simulink model "Force_Cotrol_Test"  (R2020a)
settings: Solver=FixedStepAuto  StartTime=0.0  StopTime=inf  FixedStep=0.002  RelTol=1e-3  EnableMultiTasking=on
libraries: xpcethercatlib x8, slrtlib x6, simulink x2, simulink_extras x1
settings Model: xpc_rtwmakecfg_data=_xpcethercatlib_  SimulationMode=external  Creator=Ali  LastModifiedBy=Ali
settings SolverCC: ConcurrentTasks=on  AutoInsertRateTranBlk=on
settings DataIOCC: SaveFormat=StructureWithTime
settings OptimizationCC: BlockReduction=off  OptimizeBlockIOStorage=off
settings HardwareCC: ProdBitPerPointer=32  ProdBitPerSizeT=32  ProdBitPerPtrDiffT=32  ProdLargestAtomicFloat=None  ProdWordSize=32  ProdLongLongMode=on  ProdHWDeviceType=Generic->32-bit x86 compatible
settings RTWCC: Description=Simulink Real-Time  SystemTargetFile=slrt.tlc  TemplateMakefile=slrt_default_tmf  CodeExecutionProfiling=on  CodeProfilingInstrumentation=detailed  RTWCompilerOptimization=on
settings SimulinkRealTimeCC: SupportVariableSizeSignals=on  xPCConcurrentTasks=on

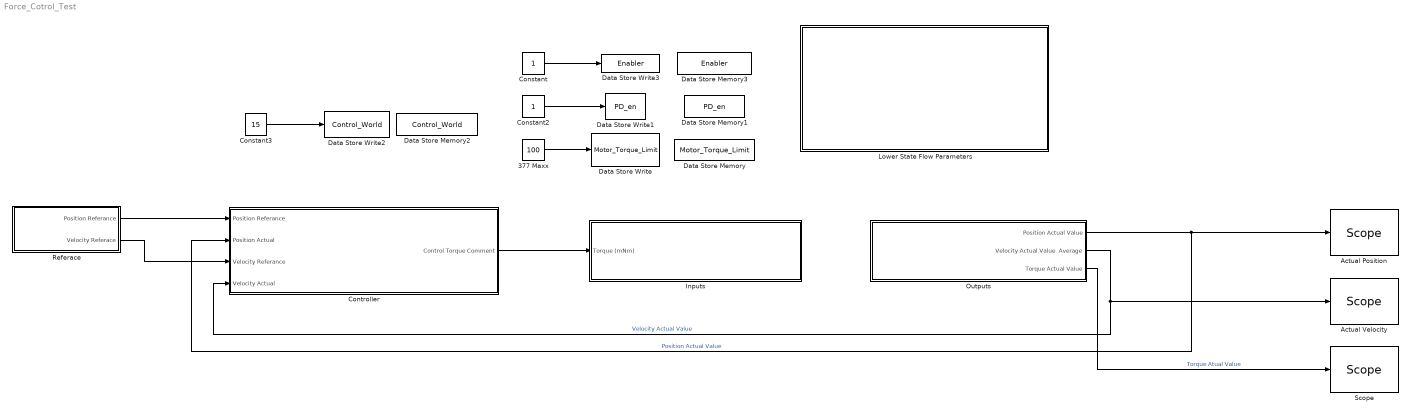
== system Force_Cotrol_Test ==
  377 Maxx : Constant  Value=100
  "Actual Position " : slrtlib/Displays and Logging/Scope   scopeno=4  scopetype=Target  autostart=on  viewmode=Graphical redraw  formatstr='%15.6f'  grid=on  ylimits=[0,0]  nosamples=250  noprepostsamples=0  interleave=1  triggermode=FreeRun  triggersignal=1  trigsignalfromport=off  triggerlevel=0.0  triggerslope=Either  triggerscope=1  triggersample=0  filename=data.dat  mode=Lazy  writesize=512  autorestart=off  dynamicfilemode=off  maxwritefilesize=512*1024^2
  Actual Velocity : slrtlib/Displays and Logging/Scope   scopeno=5  scopetype=Target  autostart=on  viewmode=Graphical redraw  formatstr='%15.6f'  grid=on  ylimits=[0,0]  nosamples=250  noprepostsamples=0  interleave=1  triggermode=FreeRun  triggersignal=1  trigsignalfromport=off  triggerlevel=0.0  triggerslope=Either  triggerscope=1  triggersample=0  filename=data.dat  mode=Lazy  writesize=512  autorestart=off  dynamicfilemode=off  maxwritefilesize=512*1024^2
  Constant : Constant
  Constant2 : Constant
  Constant3 : Constant  Value=15
  Controller : Subsystem
  Data Store Memory : DataStoreMemory  DataStoreName=Motor_Torque_Limit  ReadBeforeWriteMsg=warning  WriteAfterWriteMsg=warning  WriteAfterReadMsg=warning  ShowAdditionalParam=off
  Data Store Memory1 : DataStoreMemory  DataStoreName=PD_en  ReadBeforeWriteMsg=warning  WriteAfterWriteMsg=warning  WriteAfterReadMsg=warning  ShowAdditionalParam=off
  Data Store Memory2 : DataStoreMemory  DataStoreName=Control_World  ReadBeforeWriteMsg=warning  WriteAfterWriteMsg=warning  WriteAfterReadMsg=warning  ShowAdditionalParam=off
  Data Store Memory3 : DataStoreMemory  DataStoreName=Enabler  ReadBeforeWriteMsg=warning  WriteAfterWriteMsg=warning  WriteAfterReadMsg=warning  ShowAdditionalParam=off
  Data Store Write : DataStoreWrite  DataStoreName=Motor_Torque_Limit
  Data Store Write1 : DataStoreWrite  DataStoreName=PD_en
  Data Store Write2 : DataStoreWrite  DataStoreName=Control_World
  Data Store Write3 : DataStoreWrite  DataStoreName=Enabler
  Inputs : Subsystem
  Lower State Flow Parameters : Subsystem
  Outputs : Subsystem
  Referace : Subsystem
  "Scope " : slrtlib/Displays and Logging/Scope   scopeno=6  scopetype=Target  autostart=on  viewmode=Graphical redraw  formatstr='%15.6f'  grid=on  ylimits=[0,0]  nosamples=250  noprepostsamples=0  interleave=1  triggermode=FreeRun  triggersignal=1  trigsignalfromport=off  triggerlevel=0.0  triggerslope=Either  triggerscope=1  triggersample=0  filename=data.dat  mode=Lazy  writesize=512  autorestart=off  dynamicfilemode=off  maxwritefilesize=512*1024^2
  wires:
  377 Maxx/1 -> Data Store Write/1
  Outputs/1(Position Actual Value) -> Controller/2("Position Actual "), "Actual Position "/1  "Position Actual Value"
  Outputs/2(Velocity Actual Value  Average) -> Controller/4(Velocity Actual), Actual Velocity/1  "Velocity Actual Value"
  Referace/1(Position Referance) -> Controller/1(Position Referance)
  Referace/2(Velocity Referace) -> Controller/3(Velocity Referance)
  Constant2/1 -> Data Store Write1/1
  Controller/1(Control Torque Comment) -> Inputs/1(Torque (mNm))
  Constant3/1 -> Data Store Write2/1
  Constant/1 -> Data Store Write3/1
  Outputs/3(Torque Actual Value) -> "Scope "/1  "Torque Atual Value"

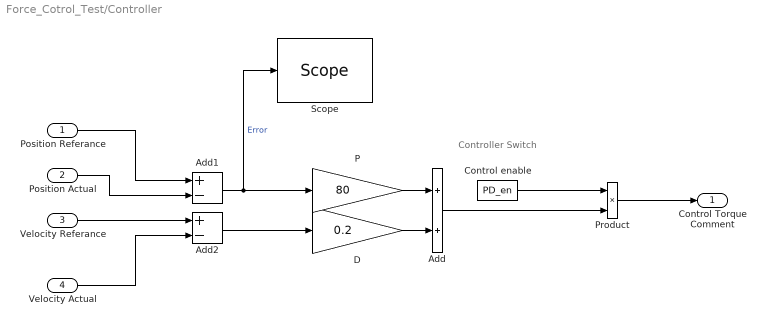
== system Force_Cotrol_Test/Controller ==
  note: Controller Switch
  Position Referance : Inport
  "Position Actual " : Inport  Port=2
  Velocity Referance : Inport  Port=3
  Velocity Actual : Inport  Port=4
  Add : Sum
  Add1 : Sum  Inputs=+-
  Add2 : Sum  Inputs=+-
  Control enable : DataStoreRead  DataStoreName=PD_en
  D : Gain  Gain=0.2
  P : Gain  Gain=80
  Product : Product
  "Scope " : slrtlib/Displays and Logging/Scope   scopeno=2  scopetype=Target  autostart=on  viewmode=Graphical redraw  formatstr='%15.6f'  grid=on  ylimits=[0,0]  nosamples=250  noprepostsamples=0  interleave=1  triggermode=FreeRun  triggersignal=1  trigsignalfromport=off  triggerlevel=0.0  triggerslope=Either  triggerscope=1  triggersample=0  filename=data.dat  mode=Lazy  writesize=512  autorestart=off  dynamicfilemode=off  maxwritefilesize=512*1024^2
  Control Torque Comment : Outport
  wires:
  D/1 -> Add/2
  Add2/1 -> D/1
  Product/1 -> Control Torque Comment/1
  Add1/1 -> "Scope "/1, P/1  "Error"
  Add/1 -> Product/2
  Velocity Referance/1 -> Add2/1
  "Position Actual "/1 -> Add1/2
  Position Referance/1 -> Add1/1
  P/1 -> Add/1
  Velocity Actual/1 -> Add2/2
  Control enable/1 -> Product/1

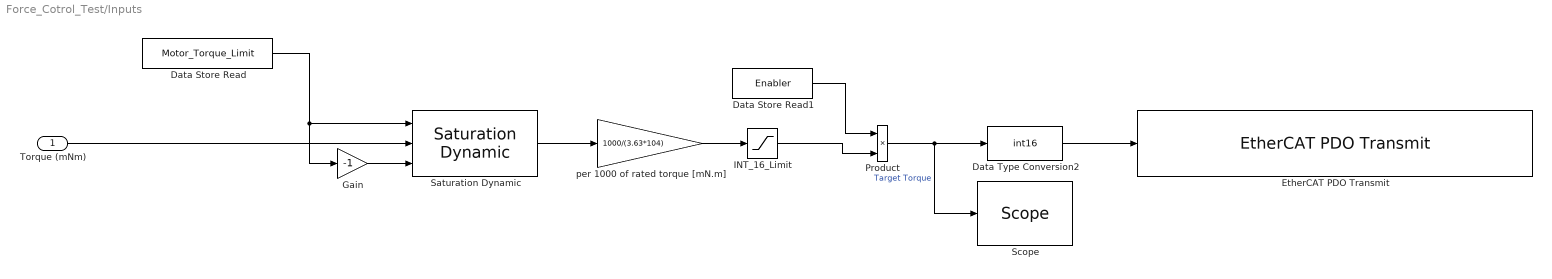
== system Force_Cotrol_Test/Inputs ==
  Torque (mNm) : Inport
  Data Store Read : DataStoreRead  DataStoreName=Motor_Torque_Limit
  Data Store Read1 : DataStoreRead  DataStoreName=Enabler
  Data Type Conversion2 : DataTypeConversion  OutDataTypeStr=int16
  "EtherCAT PDO Transmit " : xpcethercatlib/EtherCAT PDO Transmit   Priority=3  sig_name=Drive 1 (EPOS4).Module 1 (CST Mode).CST Outputs.Target torque  sig_offset=584  sig_type=int16  type_size=16  sig_dim=1  device_id=0  sample_time=0.002000
      settings: SourceProductBaseCode=XP
  Gain : Gain  Gain=-1
  INT_16_Limit : Saturate  UpperLimit=2^15-1  LowerLimit=-2^15-1
  Product : Product
  Saturation Dynamic : simulink/Discontinuities/Saturation Dynamic  OutMin=[]  OutMax=[]  OutDataTypeStr=Inherit: Same as second input  OutDataType=fixdt(1, 16)  OutScaling=2^-10  DoSatur=off
  "Scope " : slrtlib/Displays and Logging/Scope   scopeno=3  scopetype=Target  autostart=on  viewmode=Graphical redraw  formatstr='%15.6f'  grid=on  ylimits=[0,0]  nosamples=250  noprepostsamples=0  interleave=1  triggermode=FreeRun  triggersignal=1  trigsignalfromport=off  triggerlevel=0.0  triggerslope=Either  triggerscope=1  triggersample=0  filename=data.dat  mode=Lazy  writesize=512  autorestart=off  dynamicfilemode=off  maxwritefilesize=512*1024^2
  per 1000 of rated torque [mN.m] : Gain  Gain=1000/(3.63*104)  OutDataTypeStr=double
  wires:
  per 1000 of rated torque [mN.m]/1 -> INT_16_Limit/1
  Torque (mNm)/1 -> Saturation Dynamic/2
  Saturation Dynamic/1 -> per 1000 of rated torque [mN.m]/1
  Gain/1 -> Saturation Dynamic/3
  Data Store Read/1 -> Gain/1, Saturation Dynamic/1
  Data Type Conversion2/1 -> "EtherCAT PDO Transmit "/1
  Data Store Read1/1 -> Product/1
  Product/1 -> "Scope "/1, Data Type Conversion2/1  "Target Torque"
  INT_16_Limit/1 -> Product/2

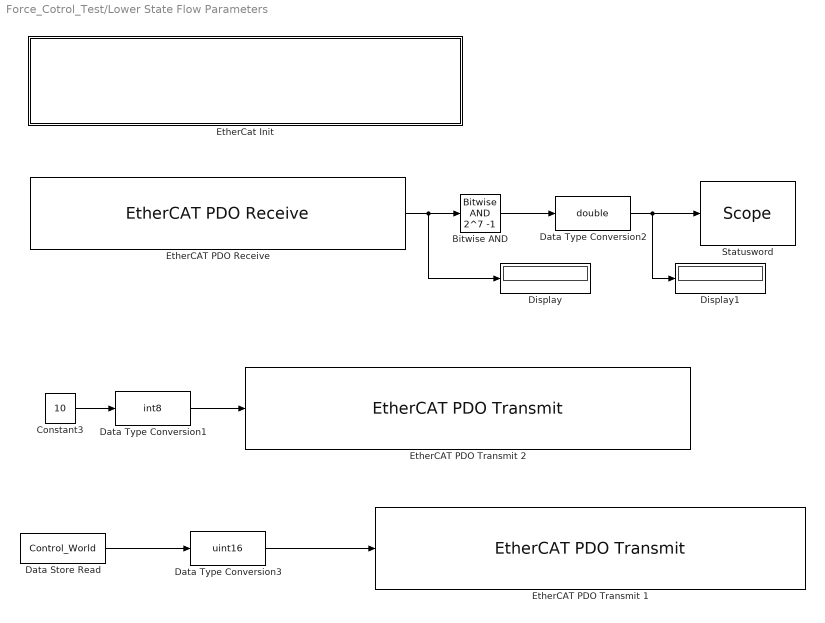
== system Force_Cotrol_Test/Lower State Flow Parameters ==
  Bitwise AND : simulink/Logic and Bit Operations/Bitwise Operator  logicop=AND  UseBitMask=on  BitMask=2^7 -1  BitMaskRealWorld=Stored Integer
  Constant3 : Constant  Value=10
  Data Store Read : DataStoreRead  DataStoreName=Control_World
  Data Type Conversion1 : DataTypeConversion  OutDataTypeStr=int8
  Data Type Conversion2 : DataTypeConversion  OutDataTypeStr=double
  Data Type Conversion3 : DataTypeConversion  OutDataTypeStr=uint16
  Display : Display
  Display1 : Display
  EtherCAT PDO Receive : xpcethercatlib/EtherCAT PDO Receive  Priority=2  sig_name=Drive 1 (EPOS4).Module 1 (CST Mode).CST Inputs.Statusword  sig_offset=568  sig_type=uint16  type_size=16  sig_dim=1  device_id=0  sample_time=0.002000
      settings: SourceProductBaseCode=XP
  EtherCAT PDO Transmit 1 : xpcethercatlib/EtherCAT PDO Transmit   Priority=3  sig_name=Drive 1 (EPOS4).Module 1 (CST Mode).CST Outputs.Controlword  sig_offset=568  sig_type=uint16  type_size=16  sig_dim=1  device_id=0  sample_time=0.002000
      settings: SourceProductBaseCode=XP
  EtherCAT PDO Transmit 2 : xpcethercatlib/EtherCAT PDO Transmit   Priority=3  sig_name=Drive 1 (EPOS4).Module 1 (CST Mode).CST Outputs.Mode of operation  sig_offset=600  sig_type=int8  type_size=8  sig_dim=1  device_id=0  sample_time=0.002000
      settings: SourceProductBaseCode=XP
  EtherCat Init : Subsystem
  Statusword : slrtlib/Displays and Logging/Scope   scopeno=1  scopetype=Target  autostart=on  viewmode=Graphical redraw  formatstr='%15.6f'  grid=on  ylimits=[0,0]  nosamples=250  noprepostsamples=0  interleave=1  triggermode=FreeRun  triggersignal=1  trigsignalfromport=off  triggerlevel=0.0  triggerslope=Either  triggerscope=1  triggersample=0  filename=data.dat  mode=Lazy  writesize=512  autorestart=off  dynamicfilemode=off  maxwritefilesize=512*1024^2
  wires:
  Bitwise AND/1 -> Data Type Conversion2/1
  Constant3/1 -> Data Type Conversion1/1
  EtherCAT PDO Receive/1 -> Display/1, Bitwise AND/1
  Data Type Conversion1/1 -> EtherCAT PDO Transmit 2/1
  Data Type Conversion2/1 -> Display1/1, Statusword/1
  Data Store Read/1 -> Data Type Conversion3/1
  Data Type Conversion3/1 -> EtherCAT PDO Transmit 1/1

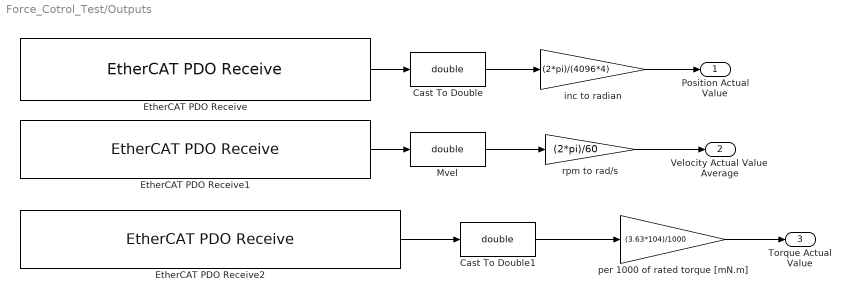
== system Force_Cotrol_Test/Outputs ==
  Cast To Double : DataTypeConversion  OutDataTypeStr=double
  Cast To Double1 : DataTypeConversion  OutDataTypeStr=double
  EtherCAT PDO Receive : xpcethercatlib/EtherCAT PDO Receive  Priority=2  sig_name=Drive 1 (EPOS4).Module 1 (CST Mode).CST Inputs.Position actual value  sig_offset=584  sig_type=int32  type_size=32  sig_dim=1  device_id=0  sample_time=0.002000
      settings: SourceProductBaseCode=XP
  EtherCAT PDO Receive1 : xpcethercatlib/EtherCAT PDO Receive  Priority=2  sig_name=Drive 1 (EPOS4).Module 1 (CST Mode).CST Inputs.Velocity actual value averaged  sig_offset=680  sig_type=int32  type_size=32  sig_dim=1  device_id=0  sample_time=0.002000
      settings: SourceProductBaseCode=XP
  EtherCAT PDO Receive2 : xpcethercatlib/EtherCAT PDO Receive  Priority=2  sig_name=Drive 1 (EPOS4).Module 1 (CST Mode).CST Inputs.Torque actual value  sig_offset=648  sig_type=int16  type_size=16  sig_dim=1  device_id=0  sample_time=0.002000
      settings: SourceProductBaseCode=XP
  Mvel : DataTypeConversion  OutDataTypeStr=double
  inc to radian : Gain  Gain=(2*pi)/(4096*4)
  per 1000 of rated torque [mN.m] : Gain  Gain=(3.63*104)/1000  OutDataTypeStr=double
  rpm to rad/s : Gain  Gain=(2*pi)/60
  Position Actual Value : Outport
  Velocity Actual Value  Average : Outport  Port=2
  Torque Actual Value : Outport  Port=3
  wires:
  Cast To Double/1 -> inc to radian/1
  EtherCAT PDO Receive/1 -> Cast To Double/1
  inc to radian/1 -> Position Actual Value/1
  EtherCAT PDO Receive1/1 -> Mvel/1
  Mvel/1 -> rpm to rad/s/1
  rpm to rad/s/1 -> Velocity Actual Value  Average/1
  per 1000 of rated torque [mN.m]/1 -> Torque Actual Value/1
  Cast To Double1/1 -> per 1000 of rated torque [mN.m]/1
  EtherCAT PDO Receive2/1 -> Cast To Double1/1

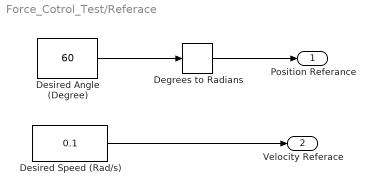
== system Force_Cotrol_Test/Referace ==
  Degrees to Radians : simulink_extras/Transformations/Degrees to Radians
  Desired Angle (Degree) : Constant  Value=60
  Desired Speed (Rad/s) : Constant  Value=0.1
  Position Referance : Outport
  Velocity Referace : Outport  Port=2
  wires:
  Desired Angle (Degree)/1 -> Degrees to Radians/1
  Degrees to Radians/1 -> Position Referance/1
  Desired Speed (Rad/s)/1 -> Velocity Referace/1

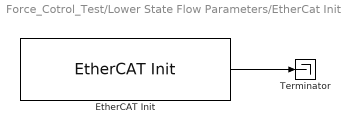
== system Force_Cotrol_Test/Lower State Flow Parameters/EtherCat Init ==
  "EtherCAT Init " : xpcethercatlib/EtherCAT Init   Priority=0  config_file=C:\Users\Ali\Desktop\Wrist_Control_Test\XML_Config_File\Test_v2_ForceControl.xml  device_id=0  pci_bus=2  pci_slot=0  pci_function=0  initstate=2  dctuning=0  enaDebug=off  enaDC=on  errLink=off  masterDbg=off  stateChgDbg=off  baseClock=off  masterCfg=off  logFile='c:\dbglog.txt'  sample_time=0.002000  DCMode=2
      settings: SourceProductBaseCode=XP
  Terminator : Terminator
  wires:
  "EtherCAT Init "/1 -> Terminator/1
